simulink model "ControllerLearningEmulation"  (R2018b)
settings: configuration reference "Active" (kept outside this file)
undefined symbols (not defined in the file): TUMHealthStatus
settings Model: DataDictionary=ControllerLearningEmulation.sldd  Creator=wischnewski  LastModifiedBy=ge34qer

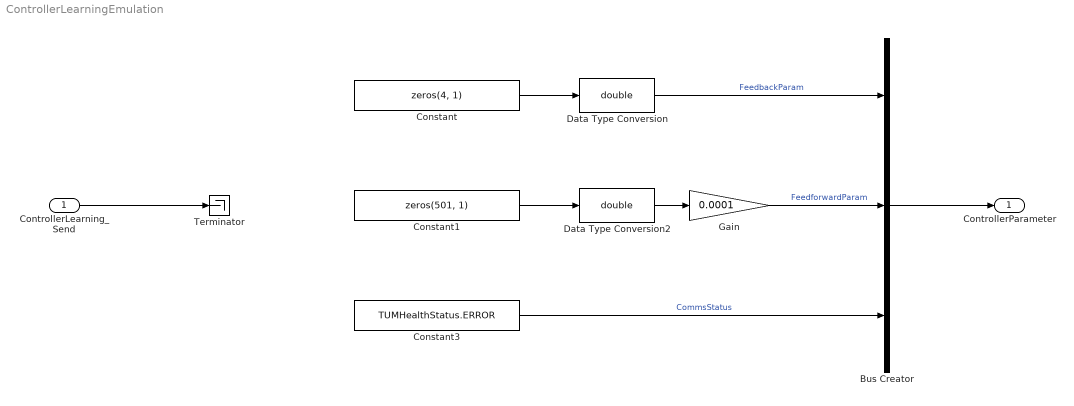
== system ControllerLearningEmulation ==
  ControllerLearning_Send : Inport  OutDataTypeStr=Bus: ControllerLearning_Send
  Bus Creator : BusCreator  Inputs=3
  Constant : Constant  Value=zeros(4, 1)
  Constant1 : Constant  Value=zeros(501, 1)
  Constant3 : Constant  Value=TUMHealthStatus.ERROR
  Data Type Conversion : DataTypeConversion  OutDataTypeStr=double
  Data Type Conversion2 : DataTypeConversion  OutDataTypeStr=double
  Gain : Gain  Gain=0.0001
  Terminator : Terminator
  ControllerParameter : Outport  OutDataTypeStr=Bus: ControllerParameter
  wires:
  Data Type Conversion2/1 -> Gain/1
  Constant1/1 -> Data Type Conversion2/1
  Constant/1 -> Data Type Conversion/1
  Constant3/1 -> Bus Creator/3  "CommsStatus"
  Gain/1 -> Bus Creator/2  "FeedforwardParam"
  Bus Creator/1 -> ControllerParameter/1
  Data Type Conversion/1 -> Bus Creator/1  "FeedbackParam"
  ControllerLearning_Send/1 -> Terminator/1
